simulink model "MOD5"  (R2020b)
settings: Solver=VariableStepAuto  StartTime=0.0  StopTime=inf  RelTol=1e-3
settings Model: EnablePacing=on  Creator=shivanshu shukla  LastModifiedBy=shivanshu shukla

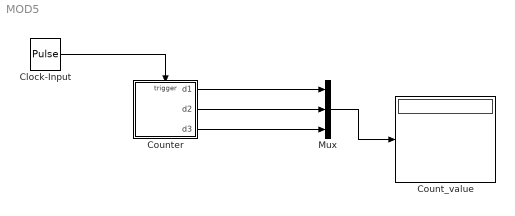
== system MOD5 ==
  Clock-Input : DiscretePulseGenerator  PulseType=Time based  Period=1  PulseWidth=2
  Count_value : Display
  Counter : Stateflow chart  TreatAsAtomicUnit=on
  Mux : Mux  Inputs=3
  wires:
  Clock-Input/1 -> Counter/Trigger
  Counter/1(d1) -> Mux/1
  Counter/2(d2) -> Mux/2
  Counter/3(d3) -> Mux/3
  Mux/1 -> Count_value/1

== stateflow chart MOD5/Counter ==
  state digit1 [parallel]
    settings: executionOrder=1
    state One
      en:
      d1=1;
    state Two
      en:
      d1=2;
    state Three
      en:
      d1=3;
    state Zero
      en:
      d1=0;
    state Four
      en:
      d1=4;
    digit1.Three -> digit1.Four : inputclk
    digit1.Zero -> digit1.One : inputclk
    digit1.One -> digit1.Two : inputclk
    digit1.Two -> digit1.Three : inputclk
    (default) -> digit1.Zero
    digit1.Four -> digit1.Zero : inputclk/{digit2.inc2;}
  state digit2 [parallel]
    settings: executionOrder=2
    state One
      en:
      d2=1;
    state Two
      en:
      d2=2;
    state Three
      en:
      d2=3;
    state Zero
      en:
      d2=0;
    state Four
      en:
      d2=4;
    digit2.Three -> digit2.Four : inc2
    digit2.Zero -> digit2.One : inc2
    digit2.One -> digit2.Two : inc2
    digit2.Two -> digit2.Three : inc2
    (default) -> digit2.Zero
    digit2.Four -> digit2.Zero : inc2/{digit3.inc3;}
  state digit3 [parallel]
    settings: executionOrder=3
    state One
      en:
      d3=1;
    state Two
      en:
      d3=2;
    state Three
      en:
      d3=3;
    state Zero
      en:
      d3=0;
    state Four
      en:
      d3=4;
    digit3.Three -> digit3.Four : inc3
    digit3.Zero -> digit3.One : inc3
    digit3.One -> digit3.Two : inc3
    digit3.Two -> digit3.Three : inc3
    (default) -> digit3.Zero
    digit3.Four -> digit3.Zero : inc3
  data: d1 output; d2 output; d3 output
  events: inc2 local FUNCTION_CALL_EVENT; inc3 local FUNCTION_CALL_EVENT; inputclk input RISING_EDGE_EVENT
